simulink model "servo_test"  (R2020b)
settings: Solver=VariableStepDiscrete  StartTime=0.0  StopTime=10.0  MaxStep=0.001  RelTol=1e-3
values from neighbouring files (symbols this model uses):
  Gtd = c2d(Gt,T,'Tustin')    [demo.m]    (also in pendulo_modelo.m)
  Robs = [1 0 ... (first row only)    [demo.m]    (also in pendulo_modelo.m)
undefined symbols (not defined in the file or in its folder): DiscIntNeverNeededParam, Discrete, Kservo2, Time
libraries: ctrlSharedLib x1
settings Model: Creator=aleca  LastModifiedBy=aleca

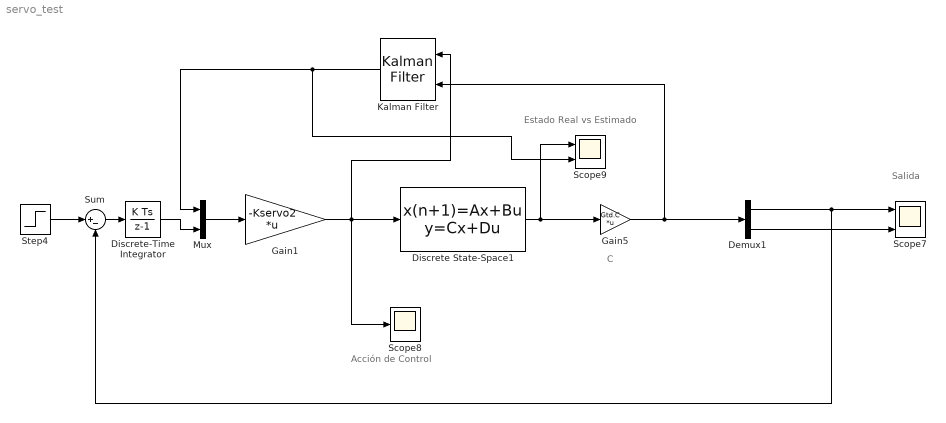
== system servo_test ==
  note: C
  note: Acción de Control
  note: Estado Real vs Estimado
  note: Salida
  Demux1 : Demux  Outputs=2
  Discrete State-Space1 : DiscreteStateSpace  A=Gtd.A  B=Gtd.B  C=eye(4)  D=zeros(4,1)  InitialCondition=[0.1 0 -0.05 0.1]  SampleTime=-1
  Discrete-Time Integrator : DiscreteIntegrator  SampleTime=-1  ICPrevOutput=DiscIntNeverNeededParam  ICPrevScaledInput=DiscIntNeverNeededParam
  Gain1 : Gain  Gain=-Kservo2  Multiplication=Matrix(K*u)
  Gain5 : Gain  Gain=Gtd.C  Multiplication=Matrix(K*u)
  Kalman Filter : ctrlSharedLib/Kalman Filter  TimeDomain=Discrete-Time  UseCurrentEstimator=off  ModelSource=Individual A, B, C, D matrices  ModelSourceVariable=ss(0.95,1,1,0,1)  A=Gtd.A  B=Gtd.B  C=Gtd.C  D=Gtd.D  NumberOfStates=1  NumberOfInputs=1  NumberOfOutputs=1  InitialEstimateSource=Dialog  X0=0  P0=10  UseK=off  UseGH=off  NumberOfProcessNoiseInputs=1  G=1  TimeInvariantG=on  H=0  TimeInvariantH=on  Q=Qobs  TimeInvariantQ=on  R=Robs  TimeInvariantR=on  N=0  TimeInvariantN=on  AddInputPort=on  AddEnablePort=off  OutputEstimatedY=off  OutputP=off  Ts=-1
  Mux : Mux  Inputs=2
  Scope7 : Scope  NumInputPorts=2
  Scope8 : Scope
  Scope9 : Scope  NumInputPorts=2
  Step4 : Step  After=-0.15  SampleTime=0.001
  Sum : Sum  Inputs=|+-
  wires:
  Discrete State-Space1/1 -> Scope9/1, Gain5/1
  Demux1/2 -> Scope7/2
  Gain5/1 -> Demux1/1, Kalman Filter/2
  Kalman Filter/1 -> Mux/1, Scope9/2
  Gain1/1 -> Kalman Filter/1, Scope8/1, Discrete State-Space1/1
  Demux1/1 -> Sum/2, Scope7/1
  Step4/1 -> Sum/1
  Mux/1 -> Gain1/1
  Discrete-Time Integrator/1 -> Mux/2
  Sum/1 -> Discrete-Time Integrator/1
